simulink model "TestMultirotorSimPx4v1_8"  (R2018b)
settings: Solver=VariableStepAuto  StartTime=0.0  StopTime=Simulation.T_END  MaxStep=Simulation.TS_MAX  RelTol=1e-3  EnableMultiTasking=on
PreLoadFcn:
  | % InitializeParameters;
undefined symbols (not defined in the file): Aero, armed, ctrl_state, Initial, Motor, Simulation, Uav, v_att_sp, v_control_mode
libraries: QuaternionLibrary x13, simulink_extras x9, Px4Library x3, dspsigattribs x1, dspstat3 x1, simulink x1
(part 9 of 9)

== matlab function TestMultirotorSimPx4v1_8/Sensor Model/Accelerometer1/Quaternion to Rotation Matrix/MATLAB Function ==
  data: q input; R output
function R = QuatToRot( q )
%QUATTOROT Convert quaternion to rotation matrix
%   Written by:    J.X.J. Bannwarth, 2017/03/27
%   Last modified: J.X.J. Bannwarth, 2018/12/11
    W = q(1);
    X = q(2);
    Y = q(3);
    Z = q(4);
    
    xx = X * X;
    xy = X * Y;
    xz = X * Z;
    xw = X * W;

    yy = Y * Y;
    yz = Y * Z;
    yw = Y * W;
    
    zz = Z * Z;
    zw = Z * W;

    m00 = 1 - 2 * ( yy + zz );
    m01 =     2 * ( xy - zw );
    m02 =     2 * ( xz + yw );

    m10 =     2 * ( xy + zw );
    m11 = 1 - 2 * ( xx + zz );
    m12 =     2 * ( yz - xw );

    m20 =     2 * ( xz - yw );
    m21 =     2 * ( yz + xw );
    m22 = 1 - 2 * ( xx + yy );
    
    R = [m00 m01 m02;
         m10 m11 m12;
         m20 m21 m22];   
end

== matlab function TestMultirotorSimPx4v1_8/att_mixerInput/Quaternion to Euler Angles2/MATLAB Function ==
  data: quat input; eul output
function eul   = QuaternionToEuler( quat )
%QUATERNIONTOEULER Convert quaternion to euler angles
%   Based on PX4 Firmware code: https://github.com/PX4/Firmware
%   Written by:    J.X.J. Bannwarth, 2016/08/29
%   Last modified: J.X.J. Bannwarth, 2018/12/11

    eul = [ atan2(2.0 .* (quat(1) .* quat(2) + quat(3) .* quat(4)), ...
                1.0 - 2.0 .* (quat(2) .* quat(2) + quat(3) .* quat(3)));
	        asin(2.0 .* (quat(1) .* quat(3) - quat(4) .* quat(2)));
            atan2(2.0 .* (quat(1) .* quat(4) + quat(2) .* quat(3)), ...
                1.0 - 2.0 .* (quat(3) .* quat(3) + quat(4) .* quat(4))) ];
end
